simulink model "actuator_controller_outer"  (R2021b)
settings: Solver=VariableStepAuto  StartTime=0.0  StopTime=20  RelTol=1e-3
values from neighbouring files (symbols this model uses):
  K_inner_act = K_inner*0.05    [analyze_actuator_control.m]
  K_outer = [0, 0, 0, 0]    [analyze_actuator_control.m]
libraries: simulink_extras x4
settings Model: Creator=austm  LastModifiedBy=austm

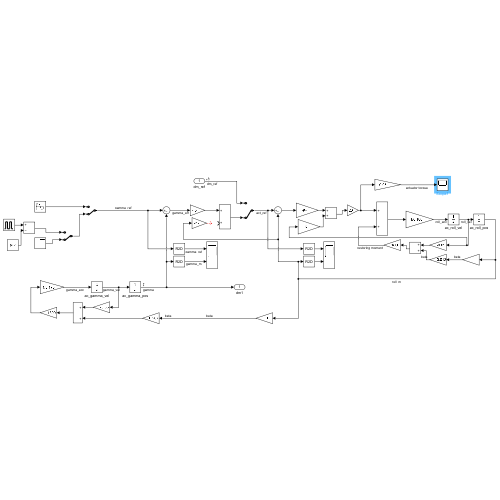
[thumbnail: Simulink's stored preview of the top-level diagram]
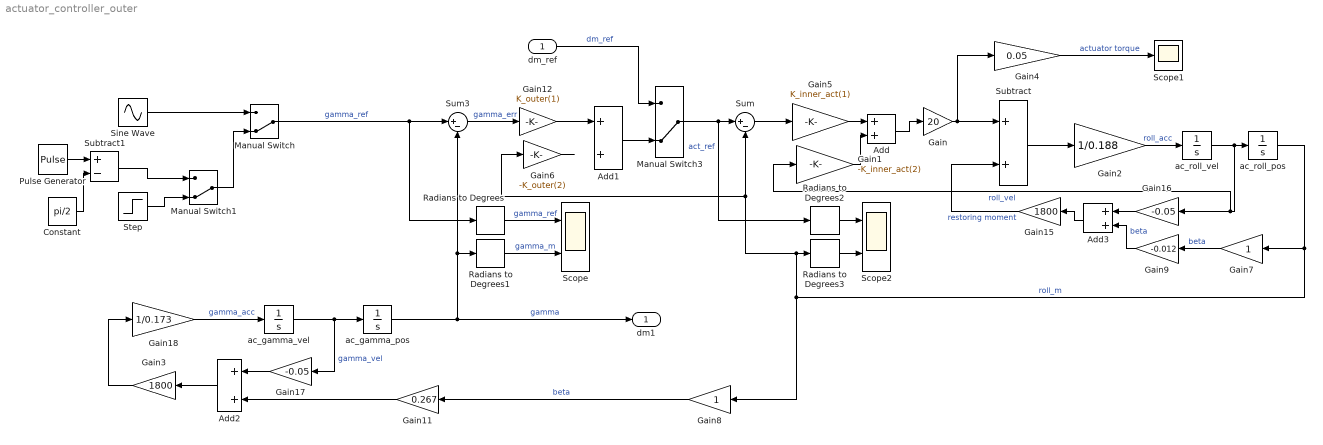
== system actuator_controller_outer ==
  dm_ref : Inport
  Add{,1..3} (4 alike) : Sum
  Constant : Constant  Value=pi/2
  Gain : Gain  Gain=20
  Gain1 : Gain  Gain=-K_inner_act(2)
  Gain11 : Gain  Gain=0.267
  Gain12 : Gain  Gain=K_outer(1)
  Gain15 : Gain  Gain=1800
  Gain16 : Gain  Gain=-0.05
  Gain17 : Gain  Gain=-0.05
  Gain18 : Gain  Gain=1/0.173
  Gain2 : Gain  Gain=1/0.188
  Gain3 : Gain  Gain=1800
  Gain4 : Gain  Gain=0.05
  Gain5 : Gain  Gain=K_inner_act(1)
  Gain6 : Gain  Gain=-K_outer(2)
  Gain7 : Gain
  Gain8 : Gain
  Gain9 : Gain  Gain=-0.012
  Manual Switch : ManualSwitch  CurrentSetting=0
  Manual Switch1 : ManualSwitch  CurrentSetting=0
  Manual Switch3 : ManualSwitch  CurrentSetting=0
  Pulse Generator : DiscretePulseGenerator  PulseType=Time based  Amplitude=pi  Period=20  PulseWidth=50
  Radians to Degrees{,1..3} (4 alike) : simulink_extras/Transformations/Radians to Degrees
  Scope : Scope  NumInputPorts=2
  Scope1 : Scope
  Scope2 : Scope  NumInputPorts=2
  Sine Wave : Sin  Amplitude=2  Frequency=0.4  SampleTime=0
  Step : Step  After=3  SampleTime=0
  Subtract : Sum
  Subtract1 : Sum  Inputs=+-
  Sum : Sum  Inputs=|+-
  Sum3 : Sum  Inputs=|+-
  ac_gamma_pos : Integrator  UpperSaturationLimit=100  LowerSaturationLimit=-100
  ac_gamma_vel : Integrator  UpperSaturationLimit=100  LowerSaturationLimit=-100
  ac_roll_pos : Integrator  UpperSaturationLimit=100  LowerSaturationLimit=-100
  ac_roll_vel : Integrator  UpperSaturationLimit=100  LowerSaturationLimit=-100
  dm1 : Outport
  wires:
  ac_roll_pos/1 -> Gain7/1, Gain6/1, Sum/2, Radians to Degrees3/1, Gain8/1  "roll_m"
  Gain2/1 -> ac_roll_vel/1  "roll_acc"
  Subtract/1 -> Gain2/1
  Subtract1/1 -> Manual Switch1/1
  Sine Wave/1 -> Manual Switch/1
  Step/1 -> Manual Switch1/2
  Manual Switch1/1 -> Manual Switch/2
  Sum3/1 -> Gain12/1  "gamma_err"
  Gain/1 -> Subtract/1, Gain4/1
  ac_roll_vel/1 -> Gain1/1, Gain16/1, ac_roll_pos/1  "roll_vel"
  Gain5/1 -> Add/1
  Gain8/1 -> Gain11/1  "beta"
  Gain11/1 -> Add2/2
  Gain3/1 -> Gain18/1
  ac_gamma_vel/1 -> Gain17/1, ac_gamma_pos/1  "gamma_vel"
  Gain18/1 -> ac_gamma_vel/1  "gamma_acc"
  Add2/1 -> Gain3/1
  Gain17/1 -> Add2/1
  Manual Switch/1 -> Radians to Degrees/1, Sum3/1  "gamma_ref"
  ac_gamma_pos/1 -> dm1/1, Sum3/2, Radians to Degrees1/1  "gamma"
  Pulse Generator/1 -> Subtract1/1
  Constant/1 -> Subtract1/2
  Gain12/1 -> Add1/1
  Manual Switch3/1 -> Radians to Degrees2/1, Sum/1  "act_ref"
  Radians to Degrees/1 -> Scope/1  "gamma_ref"
  Radians to Degrees1/1 -> Scope/2  "gamma_m"
  Gain4/1 -> Scope1/1  "actuator torque"
  Sum/1 -> Gain5/1
  Gain15/1 -> Subtract/2  "restoring moment"
  Radians to Degrees3/1 -> Scope2/2
  Radians to Degrees2/1 -> Scope2/1
  Gain16/1 -> Add3/1
  Add1/1 -> Manual Switch3/2
  Gain6/1 -> ?
  dm_ref/1 -> Manual Switch3/1  "dm_ref"
  Add/1 -> Gain/1
  Gain1/1 -> Add/2
  Add3/1 -> Gain15/1
  Gain7/1 -> Gain9/1  "beta"
  Gain9/1 -> Add3/2  "beta"
